simulink model "RC_circuit"  (Simulink 10.1)
settings: Solver=FixedStepAuto  StartTime=0.0  StopTime=stopTime  FixedStep=T  RelTol=1e-3
values from neighbouring files (symbols this model uses):
  C = 1e-4    (= 0.0001)    [init_RC_devresi.m]    (also in init_RC_devresi_bang_bang_kontrol.m; init_araba_hiz_kontrol.m = [0 1]; init_araba_hiz_on_off_kontrol.m = [0 1]; init_araba_hiz_pid_kontrol.m = [0 1])
  R = 3300    [init_RC_devresi.m]    (also in init_RC_devresi_bang_bang_kontrol.m = 1000)
  V0 = 0    [init_RC_devresi.m]    (also in init_RC_devresi_bang_bang_kontrol.m)
  Vcc = 5    [init_RC_devresi.m]
settings Model: Creator=TULPAR  LastModifiedBy=TULPAR
settings DataIOCC: SaveFormat=Dataset  SaveOutput=off  ReturnWorkspaceOutputs=on
settings OptimizationCC: LifeSpan=auto
settings DebuggingCC: UnderspecifiedInitializationDetection=Simplified  MergeDetectMultiDrivingBlocksExec=error  SFUnexpectedBacktrackingDiag=error  SFNoUnconditionalDefaultTransitionDiag=error  SFExecutionAtInitializationDiag=warning  ArithmeticOperatorsInVariantConditions=error
settings HardwareCC: ProdBitPerPointer=64  ProdBitPerSizeT=64  ProdBitPerPtrDiffT=64  ProdLargestAtomicFloat=Float  ProdIntDivRoundTo=Zero  ProdEndianess=LittleEndian  ProdWordSize=64  ProdHWDeviceType=Intel->x86-64 (Windows64)
settings ModelReferenceCC: PropagateSignalLabelsOutOfModel=on
settings SFSimCC: SimUseLocalCustomCode=on  CustomCodeUndefinedFunction=FilterOut
settings RTWCC: RTWUseLocalCustomCode=on
settings CodeAppCC: StateflowObjectComments=off
settings GRTTargetCC: TargetLangStandard=C99 (ISO)  CombineOutputUpdateFcns=on  GRTInterface=off
settings ConfigComp: CovMetricSettings=dwe  CovHtmlReporting=off  CovSaveCumulativeToWorkspaceVar=off  CovSaveSingleToWorkspaceVar=off  CovExternalEMLEnable=on

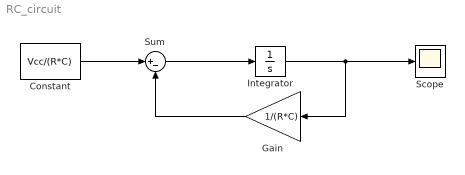
== system RC_circuit ==
  Constant : Constant  Value=Vcc/(R*C)
  Gain : Gain  Gain=1/(R*C)
  Integrator : Integrator  InitialCondition=V0
  Scope : Scope
  Sum : Sum  Inputs=|+-
  wires:
  Constant/1 -> Sum/1
  Integrator/1 -> Scope/1, Gain/1
  Gain/1 -> Sum/2
  Sum/1 -> Integrator/1
